simulink model "nonLinear_3_1_positive"  (R2021a)
settings: Solver=VariableStepAuto  StartTime=0.0  StopTime=100  RelTol=1e-3
undefined symbols (not defined in the file): b, D, g_acc, I, invA, invI, invM, Ix, Iy, Iz, k, Kd_p, Kd_r, Kd_y, Kd_z, Ki_p, Ki_r, Ki_y, Ki_z, Kp_p, Kp_r, Kp_y, Kp_z, L, m, mg
libraries: vrlib x1
settings Model: Creator=filippo  LastModifiedBy=filippo

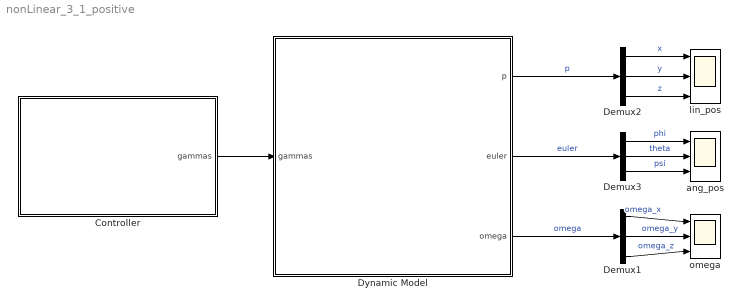
== system nonLinear_3_1_positive ==
  Controller : Subsystem
  Demux1 : Demux  Outputs=3
  Demux2 : Demux  Outputs=3
  Demux3 : Demux  Outputs=3
  Dynamic Model : Subsystem
  ang_pos : Scope  NumInputPorts=3
  lin_pos : Scope  NumInputPorts=3
  omega : Scope  NumInputPorts=3
  wires:
  Dynamic Model/2(euler) -> Demux3/1  "euler"
  Dynamic Model/1(p) -> Demux2/1  "p"
  Demux2/1 -> lin_pos/1  "x"
  Demux3/2 -> ang_pos/2  "theta"
  Demux2/3 -> lin_pos/3  "z"
  Demux2/2 -> lin_pos/2  "y"
  Demux3/3 -> ang_pos/3  "psi"
  Demux3/1 -> ang_pos/1  "phi"
  Controller/1(gammas) -> Dynamic Model/1(gammas)
  Demux1/1 -> omega/1  "omega_x"
  Demux1/3 -> omega/3  "omega_z"
  Demux1/2 -> omega/2  "omega_y"
  Dynamic Model/3(omega) -> Demux1/1  "omega"

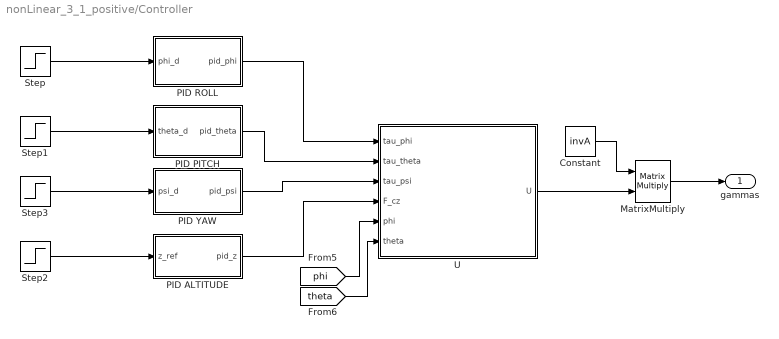
== system nonLinear_3_1_positive/Controller ==
  Constant : Constant  Value=invA
  MatrixMultiply : Product  Multiplication=Matrix(*)
  PID ALTITUDE : Subsystem
  PID PITCH : Subsystem
  PID ROLL : Subsystem
  PID YAW : Subsystem
  Step : Step  Time=0  After=0  SampleTime=0
  Step1 : Step  After=0  SampleTime=0
  Step2 : Step  Time=0  SampleTime=0
  Step3 : Step  Time=0  After=0  SampleTime=0
  U : MATLAB Function  TreatAsAtomicUnit=on
  gammas : Outport
  wires:
  PID YAW/1(pid_psi) -> U/3(tau_psi)
  [theta] -> U/6(theta)
  PID ROLL/1(pid_phi) -> U/1(tau_phi)
  [phi] -> U/5(phi)
  PID ALTITUDE/1(pid_z) -> U/4(F_cz)
  PID PITCH/1(pid_theta) -> U/2(tau_theta)
  Step2/1 -> PID ALTITUDE/1(z_ref)
  Step3/1 -> PID YAW/1(psi_d)
  Step/1 -> PID ROLL/1(phi_d)
  Step1/1 -> PID PITCH/1(theta_d)
  MatrixMultiply/1 -> gammas/1
  Constant/1 -> MatrixMultiply/1
  U/1(U) -> MatrixMultiply/2

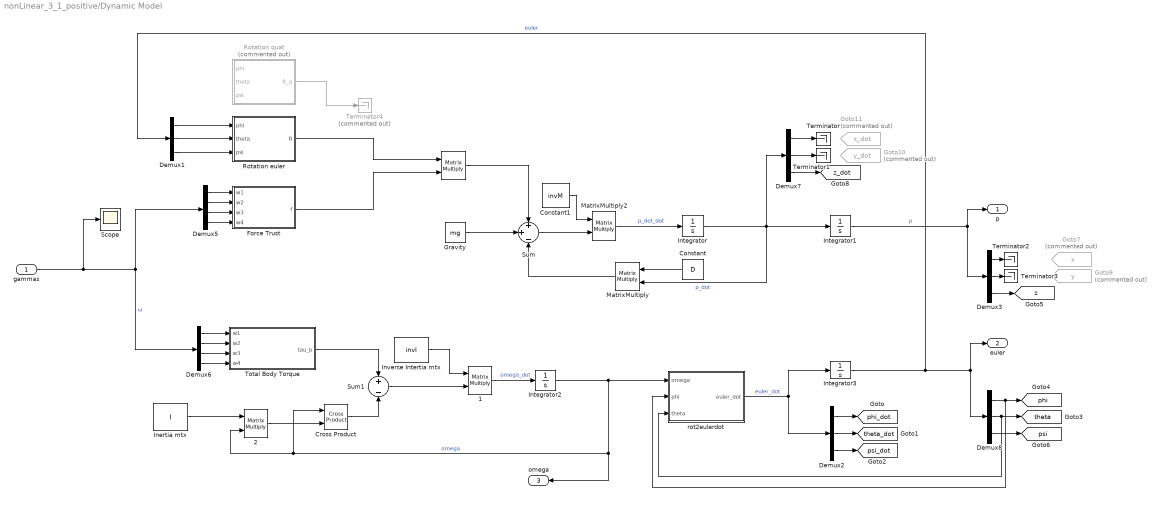
== system nonLinear_3_1_positive/Dynamic Model ==
  gammas : Inport
  " " : Product  Multiplication=Matrix(*)
  " 1" : Product  Multiplication=Matrix(*)
  " 2" : Product  Multiplication=Matrix(*)
  Constant : Constant  Value=D
  Constant1 : Constant  Value=invM
  Cross Product : vrlib/Utilities/Cross Product
  Demux{1..3,7..8} (5 alike) : Demux  Outputs=3
  Demux5 : Demux
  Demux6 : Demux
  Force Trust : MATLAB Function  TreatAsAtomicUnit=on
  Goto10 : Goto  Commented=on  GotoTag=y_dot  TagVisibility=global
  Goto11 : Goto  Commented=on  GotoTag=x_dot  TagVisibility=global
  Goto7 : Goto  Commented=on  GotoTag=x  TagVisibility=global
  Goto9 : Goto  Commented=on  GotoTag=y  TagVisibility=global
  Gravity : Constant  Value=mg  VectorParams1D=off
  Inertia mtx : Constant  Value=I  VectorParams1D=off
  Integrator{,1..3} (4 alike) : Integrator
  Inverse Intertia mtx : Constant  Value=invI
  MatrixMultiply : Product  Multiplication=Matrix(*)
  MatrixMultiply2 : Product  Multiplication=Matrix(*)
  Rotation euler : MATLAB Function  TreatAsAtomicUnit=on
  Rotation quat : MATLAB Function  Commented=on  TreatAsAtomicUnit=on
  Scope : Scope
  Sum : Sum  Inputs=+|+|-
  Sum1 : Sum  Inputs=+|-
  Terminator{,1..3} (4 alike) : Terminator
  Terminator4 : Terminator  Commented=on
  Total Body Torque : MATLAB Function  TreatAsAtomicUnit=on
  rot2eulerdot : MATLAB Function  TreatAsAtomicUnit=on
  p : Outport
  euler : Outport  Port=2
  omega : Outport  Port=3
  tag scope: phi=global, phi_dot=global, psi=global, psi_dot=global, theta=global, theta_dot=global, z=global, z_dot=global
  wires:
  " "/1 -> Sum/1
  " 2"/1 -> Cross Product/2
  Demux5/4 -> Force Trust/4(w4)
  Demux1/3 -> Rotation euler/3(psi)
  Demux5/2 -> Force Trust/2(w2)
  Gravity/1 -> Sum/2
  Demux1/1 -> Rotation euler/1(phi)
  Demux1/2 -> Rotation euler/2(theta)
  Demux6/4 -> Total Body Torque/4(w4)
  Force Trust/1(f) -> " "/2
  Demux5/3 -> Force Trust/3(w3)
  Demux6/1 -> Total Body Torque/1(w1)
  gammas/1 -> Scope/1, Demux6/1, Demux5/1  "ω"
  Integrator2/1 -> rot2eulerdot/1(omega), " 2"/2, Cross Product/1, omega/1  "omega"
  Demux6/3 -> Total Body Torque/3(w3)
  Demux5/1 -> Force Trust/1(w1)
  Demux6/2 -> Total Body Torque/2(w2)
  Demux2/1 -> [phi_dot]
  Demux2/3 -> [psi_dot]
  Demux2/2 -> [theta_dot]
  Demux3/3 -> [z]
  Integrator1/1 -> Demux3/1, p/1  "p"
  Integrator/1 -> MatrixMultiply/2, Integrator1/1, Demux7/1  "p_dot"
  Demux7/3 -> [z_dot]
  Total Body Torque/1(tau_b) -> Sum1/1
  Cross Product/1 -> Sum1/2
  " 1"/1 -> Integrator2/1  "omega_dot"
  Sum1/1 -> " 1"/2
  Inertia mtx/1 -> " 2"/1
  Inverse Intertia mtx/1 -> " 1"/1
  Constant/1 -> MatrixMultiply/1
  MatrixMultiply/1 -> Sum/3
  rot2eulerdot/1(euler_dot) -> Integrator3/1, Demux2/1  "euler_dot"
  Integrator3/1 -> Demux8/1, euler/1, Demux1/1  "euler"
  Demux8/3 -> [psi]
  Demux8/2 -> rot2eulerdot/3(theta), [theta]
  Demux8/1 -> rot2eulerdot/2(phi), [phi]
  Constant1/1 -> MatrixMultiply2/1
  MatrixMultiply2/1 -> Integrator/1  "p_dot_dot"
  Sum/1 -> MatrixMultiply2/2
  Rotation quat/1(R_q) -> Terminator4/1
  Rotation euler/1(R) -> " "/1
  Demux7/1 -> Terminator/1
  Demux7/2 -> Terminator1/1
  Demux3/1 -> Terminator2/1
  Demux3/2 -> Terminator3/1

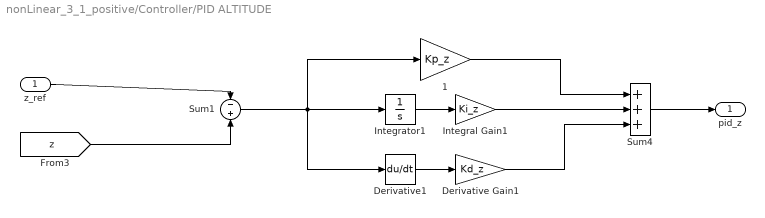
== system nonLinear_3_1_positive/Controller/PID ALTITUDE ==
  z_ref : Inport
  " 1" : Gain  Gain=Kp_z
  Derivative Gain1 : Gain  Gain=Kd_z
  Derivative1 : Derivative
  Integral Gain1 : Gain  Gain=Ki_z
  Integrator1 : Integrator
  Sum1 : Sum  Inputs=-|+
  Sum4 : Sum  Inputs=+++
  pid_z : Outport
  wires:
  Sum1/1 -> Derivative1/1, Integrator1/1, " 1"/1
  Integrator1/1 -> Integral Gain1/1
  Sum4/1 -> pid_z/1
  z_ref/1 -> Sum1/1
  " 1"/1 -> Sum4/1
  Derivative1/1 -> Derivative Gain1/1
  Derivative Gain1/1 -> Sum4/3
  [z] -> Sum1/2
  Integral Gain1/1 -> Sum4/2

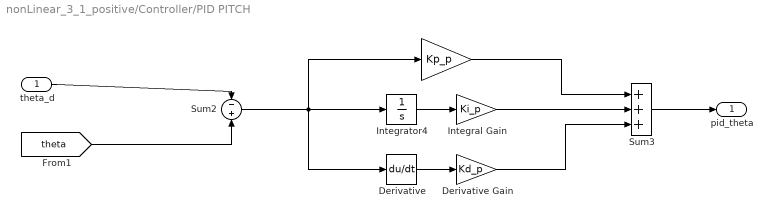
== system nonLinear_3_1_positive/Controller/PID PITCH ==
  theta_d : Inport
  " " : Gain  Gain=Kp_p
  Derivative : Derivative
  Derivative Gain : Gain  Gain=Kd_p
  Integral Gain : Gain  Gain=Ki_p
  Integrator4 : Integrator
  Sum2 : Sum  Inputs=-|+
  Sum3 : Sum  Inputs=+++
  pid_theta : Outport
  wires:
  Sum2/1 -> Derivative/1, Integrator4/1, " "/1
  Integrator4/1 -> Integral Gain/1
  Derivative/1 -> Derivative Gain/1
  " "/1 -> Sum3/1
  Integral Gain/1 -> Sum3/2
  Derivative Gain/1 -> Sum3/3
  [theta] -> Sum2/2
  Sum3/1 -> pid_theta/1
  theta_d/1 -> Sum2/1

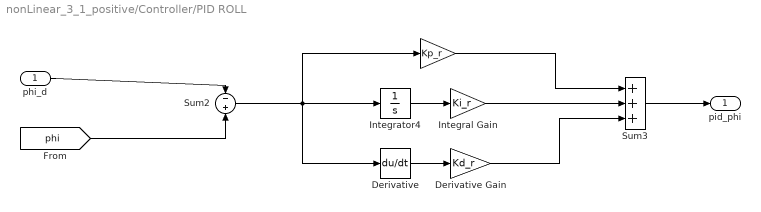
== system nonLinear_3_1_positive/Controller/PID ROLL ==
  phi_d : Inport
  " " : Gain  Gain=Kp_r
  Derivative : Derivative
  Derivative Gain : Gain  Gain=Kd_r
  Integral Gain : Gain  Gain=Ki_r
  Integrator4 : Integrator
  Sum2 : Sum  Inputs=-|+
  Sum3 : Sum  Inputs=+++
  pid_phi : Outport
  wires:
  Integrator4/1 -> Integral Gain/1
  phi_d/1 -> Sum2/1
  Sum2/1 -> Derivative/1, Integrator4/1, " "/1
  [phi] -> Sum2/2
  Derivative Gain/1 -> Sum3/3
  Integral Gain/1 -> Sum3/2
  " "/1 -> Sum3/1
  Sum3/1 -> pid_phi/1
  Derivative/1 -> Derivative Gain/1

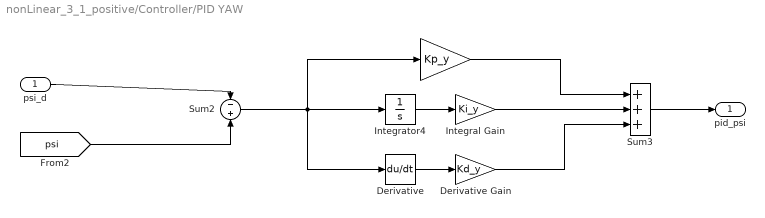
== system nonLinear_3_1_positive/Controller/PID YAW ==
  psi_d : Inport
  " " : Gain  Gain=Kp_y
  Derivative : Derivative
  Derivative Gain : Gain  Gain=Kd_y
  Integral Gain : Gain  Gain=Ki_y
  Integrator4 : Integrator
  Sum2 : Sum  Inputs=-|+
  Sum3 : Sum  Inputs=+++
  pid_psi : Outport
  wires:
  Sum2/1 -> Derivative/1, Integrator4/1, " "/1
  Integrator4/1 -> Integral Gain/1
  Sum3/1 -> pid_psi/1
  psi_d/1 -> Sum2/1
  " "/1 -> Sum3/1
  Derivative/1 -> Derivative Gain/1
  Derivative Gain/1 -> Sum3/3
  [psi] -> Sum2/2
  Integral Gain/1 -> Sum3/2

== matlab function nonLinear_3_1_positive/Dynamic Model/Force Trust ==
  data: w1 input; f output [..2]; w2 input; w3 input; w4 input; k parameter
function f = F_b(w1,w2,w3,w4,k)
mtx = k*[0; 0; w1+w2+w3+w4];
f = mtx;
end

== matlab function nonLinear_3_1_positive/Dynamic Model/Rotation euler ==
  data: phi input; R output; theta input; psi input
function R = ROTATION(phi, theta, psi)
% Rot matrix Body-fixed frame wrt Inertial frame
R = Rz(psi) * Ry(theta) * Rx(phi);
end

== matlab function nonLinear_3_1_positive/Dynamic Model/Total Body Torque ==
  data: w1 input; tau_b output; w2 input; w3 input; w4 input; L parameter; k parameter; b parameter
function tau_b= TotalBodyTorque(w1, w2, w3, w4, L, k, b)
tau_b = [L*k*(w1-w3);
         L*k*(w2-w4); 
         b*(w1-w2+w3-w4)];
end

== matlab function nonLinear_3_1_positive/Dynamic Model/Rotation quat ==
  data: phi input; R_q output; theta input; psi input
function R_q = R_QUAT(phi, theta, psi)
q = eul2quat([psi theta phi]);
R = quat2rotm(q);
end

== matlab function nonLinear_3_1_positive/Controller/U ==
  data: tau_phi input; U output; tau_theta input; tau_psi input; F_cz input; phi input; theta input; Ix parameter; Iy parameter; Iz parameter; k parameter; m parameter; g_acc parameter
function U = calcU(tau_phi, tau_theta, tau_psi,F_cz, phi, theta, Ix, Iy, Iz, k, m, g_acc)
U = [-Ix*tau_phi;
     -Iy*tau_theta;
     -Iz*tau_psi;
     m*g_acc/(k*cos(theta)*cos(phi)) + F_cz];
end

== matlab function nonLinear_3_1_positive/Dynamic Model/rot2eulerdot ==
  data: omega input; phi input; euler_dot output; theta input
function euler_dot = rot2euler(omega,phi,theta)
R = [1 0 -sin(theta); 
     0 cos(phi) cos(theta)*sin(phi);
     0 -sin(phi) cos(theta)*cos(phi)];
euler_dot = inv(R)*omega;
end
